simulink model "heat_transfer"  (R2021b)
settings: Solver=VariableStepAuto  StartTime=0.0  StopTime=10.0  RelTol=1e-3
libraries: fl_lib x21, nesl_utility x1
settings Model: Creator=310611102  LastModifiedBy=310611102

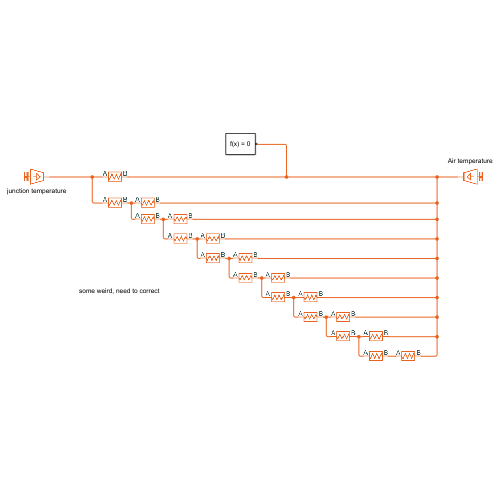
[thumbnail: Simulink's stored preview of the top-level diagram]
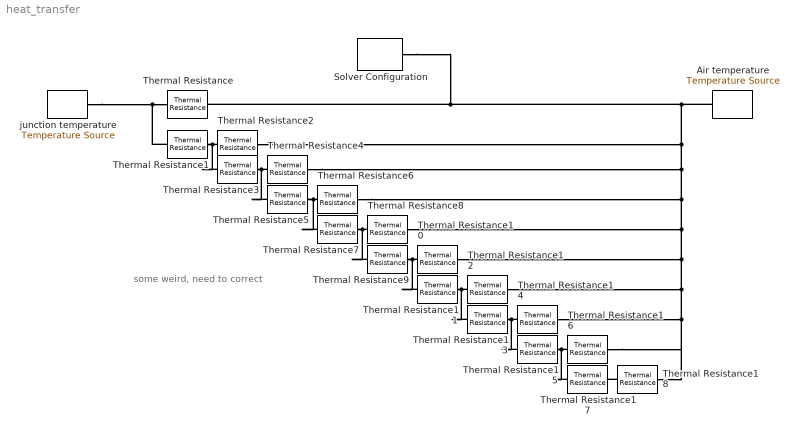
== system heat_transfer ==
  note: some weird, need to correct
  Air temperature : fl_lib/Thermal/Thermal Sources/Temperature Source  temperature=273.15+30 K
  Solver Configuration : nesl_utility/Solver Configuration  PhysicalDomain=network_engine_domain  SubClassName=solver  LeftPortType=input  RightPortType=generic  Tones=[]  Harmonics=[]  SimulateNoise=off  Profile=off  UseLocalSampling=off  EnableSwitchedLinearOptims=on  FrequencyDomain=off  UseCCode=off  RelTol=0.001  AbsTol=1e-06  MinStep=1e-09  ToWorkspace=off  RevertToSquareIcSolve=off  NumHomotopyIterations=100  PhasorMode=off  PhasorModeNumHarmonics=1  DoDC=off  ResidualTolerance=1e-09  UseLocalSolver=off  LocalSolverChoice=NE_BACKWARD_EULER_ADVANCER  LocalSolverSampleTime=0.001  DoFixedCost=off  MaxNonlinIter=3  MaxModeIter=2  ComputeImpulses=off  ImpulseIterations=2  LinearAlgebra=auto  EquationFormulation=NE_TIME_EF  DelaysMemoryBudget=1024  AutomaticFiltering=on  FilteringTimeConstant=0.001  PartitionStorageMethod=AS_NEEDED  PartitionMemoryBudget=1024  PartitionMethod=ROBUST
      settings: SourceProductBaseCode=PW,SS
  Thermal Resistance : fl_lib/Thermal/Thermal Elements/Thermal Resistance  resistance=Rchip_air K/W  T_specify=off  T_priority=None  T=0 K  T_nominal_specify=off  T_nominal_unit=K  T_nominal_value=1  Q_specify=off  Q_priority=None  Q=0 W  Q_nominal_specify=off  Q_nominal_unit=W  Q_nominal_value=1
      settings: SourceProductBaseCode=SS
  Thermal Resistance1 : fl_lib/Thermal/Thermal Elements/Thermal Resistance  resistance=Rchip_re1 K/W  T_specify=off  T_priority=None  T=0 K  T_nominal_specify=off  T_nominal_unit=K  T_nominal_value=1  Q_specify=off  Q_priority=None  Q=0 W  Q_nominal_specify=off  Q_nominal_unit=W  Q_nominal_value=1
      settings: SourceProductBaseCode=SS
  Thermal Resistance10 : fl_lib/Thermal/Thermal Elements/Thermal Resistance  resistance=Rfr45_air K/W  T_specify=off  T_priority=None  T=0 K  T_nominal_specify=off  T_nominal_unit=K  T_nominal_value=1  Q_specify=off  Q_priority=None  Q=0 W  Q_nominal_specify=off  Q_nominal_unit=W  Q_nominal_value=1
      settings: SourceProductBaseCode=SS
  Thermal Resistance11 : fl_lib/Thermal/Thermal Elements/Thermal Resistance  resistance=Rfr45_cop6 K/W  T_specify=off  T_priority=None  T=0 K  T_nominal_specify=off  T_nominal_unit=K  T_nominal_value=1  Q_specify=off  Q_priority=None  Q=0 W  Q_nominal_specify=off  Q_nominal_unit=W  Q_nominal_value=1
      settings: SourceProductBaseCode=SS
  Thermal Resistance12 : fl_lib/Thermal/Thermal Elements/Thermal Resistance  resistance=Rcop6_air K/W  T_specify=off  T_priority=None  T=0 K  T_nominal_specify=off  T_nominal_unit=K  T_nominal_value=1  Q_specify=off  Q_priority=None  Q=0 W  Q_nominal_specify=off  Q_nominal_unit=W  Q_nominal_value=1
      settings: SourceProductBaseCode=SS
  Thermal Resistance13 : fl_lib/Thermal/Thermal Elements/Thermal Resistance  resistance=Rcop6_fr47 K/W  T_specify=off  T_priority=None  T=0 K  T_nominal_specify=off  T_nominal_unit=K  T_nominal_value=1  Q_specify=off  Q_priority=None  Q=0 W  Q_nominal_specify=off  Q_nominal_unit=W  Q_nominal_value=1
      settings: SourceProductBaseCode=SS
  Thermal Resistance14 : fl_lib/Thermal/Thermal Elements/Thermal Resistance  resistance=Rfr47_air K/W  T_specify=off  T_priority=None  T=0 K  T_nominal_specify=off  T_nominal_unit=K  T_nominal_value=1  Q_specify=off  Q_priority=None  Q=0 W  Q_nominal_specify=off  Q_nominal_unit=W  Q_nominal_value=1
      settings: SourceProductBaseCode=SS
  Thermal Resistance15 : fl_lib/Thermal/Thermal Elements/Thermal Resistance  resistance=Rfr47_cop8 K/W  T_specify=off  T_priority=None  T=0 K  T_nominal_specify=off  T_nominal_unit=K  T_nominal_value=1  Q_specify=off  Q_priority=None  Q=0 W  Q_nominal_specify=off  Q_nominal_unit=W  Q_nominal_value=1
      settings: SourceProductBaseCode=SS
  Thermal Resistance16 : fl_lib/Thermal/Thermal Elements/Thermal Resistance  resistance=Rcop8_air K/W  T_specify=off  T_priority=None  T=0 K  T_nominal_specify=off  T_nominal_unit=K  T_nominal_value=1  Q_specify=off  Q_priority=None  Q=0 W  Q_nominal_specify=off  Q_nominal_unit=W  Q_nominal_value=1
      settings: SourceProductBaseCode=SS
  Thermal Resistance17 : fl_lib/Thermal/Thermal Elements/Thermal Resistance  resistance=Rcop8_re9 K/W  T_specify=off  T_priority=None  T=0 K  T_nominal_specify=off  T_nominal_unit=K  T_nominal_value=1  Q_specify=off  Q_priority=None  Q=0 W  Q_nominal_specify=off  Q_nominal_unit=W  Q_nominal_value=1
      settings: SourceProductBaseCode=SS
  Thermal Resistance18 : fl_lib/Thermal/Thermal Elements/Thermal Resistance  resistance=Rre9_air K/W  T_specify=off  T_priority=None  T=0 K  T_nominal_specify=off  T_nominal_unit=K  T_nominal_value=1  Q_specify=off  Q_priority=None  Q=0 W  Q_nominal_specify=off  Q_nominal_unit=W  Q_nominal_value=1
      settings: SourceProductBaseCode=SS
  Thermal Resistance2 : fl_lib/Thermal/Thermal Elements/Thermal Resistance  resistance=Rre1_air K/W  T_specify=off  T_priority=None  T=0 K  T_nominal_specify=off  T_nominal_unit=K  T_nominal_value=1  Q_specify=off  Q_priority=None  Q=0 W  Q_nominal_specify=off  Q_nominal_unit=W  Q_nominal_value=1
      settings: SourceProductBaseCode=SS
  Thermal Resistance3 : fl_lib/Thermal/Thermal Elements/Thermal Resistance  resistance=Rre1_cop2 K/W  T_specify=off  T_priority=None  T=0 K  T_nominal_specify=off  T_nominal_unit=K  T_nominal_value=1  Q_specify=off  Q_priority=None  Q=0 W  Q_nominal_specify=off  Q_nominal_unit=W  Q_nominal_value=1
      settings: SourceProductBaseCode=SS
  Thermal Resistance4 : fl_lib/Thermal/Thermal Elements/Thermal Resistance  resistance=Rcop2_air K/W  T_specify=off  T_priority=None  T=0 K  T_nominal_specify=off  T_nominal_unit=K  T_nominal_value=1  Q_specify=off  Q_priority=None  Q=0 W  Q_nominal_specify=off  Q_nominal_unit=W  Q_nominal_value=1
      settings: SourceProductBaseCode=SS
  Thermal Resistance5 : fl_lib/Thermal/Thermal Elements/Thermal Resistance  resistance=Rcop2_fr43 K/W  T_specify=off  T_priority=None  T=0 K  T_nominal_specify=off  T_nominal_unit=K  T_nominal_value=1  Q_specify=off  Q_priority=None  Q=0 W  Q_nominal_specify=off  Q_nominal_unit=W  Q_nominal_value=1
      settings: SourceProductBaseCode=SS
  Thermal Resistance6 : fl_lib/Thermal/Thermal Elements/Thermal Resistance  resistance=Rfr43_air K/W  T_specify=off  T_priority=None  T=0 K  T_nominal_specify=off  T_nominal_unit=K  T_nominal_value=1  Q_specify=off  Q_priority=None  Q=0 W  Q_nominal_specify=off  Q_nominal_unit=W  Q_nominal_value=1
      settings: SourceProductBaseCode=SS
  Thermal Resistance7 : fl_lib/Thermal/Thermal Elements/Thermal Resistance  resistance=Rfr43_cop4 K/W  T_specify=off  T_priority=None  T=0 K  T_nominal_specify=off  T_nominal_unit=K  T_nominal_value=1  Q_specify=off  Q_priority=None  Q=0 W  Q_nominal_specify=off  Q_nominal_unit=W  Q_nominal_value=1
      settings: SourceProductBaseCode=SS
  Thermal Resistance8 : fl_lib/Thermal/Thermal Elements/Thermal Resistance  resistance=Rcop4_air K/W  T_specify=off  T_priority=None  T=0 K  T_nominal_specify=off  T_nominal_unit=K  T_nominal_value=1  Q_specify=off  Q_priority=None  Q=0 W  Q_nominal_specify=off  Q_nominal_unit=W  Q_nominal_value=1
      settings: SourceProductBaseCode=SS
  Thermal Resistance9 : fl_lib/Thermal/Thermal Elements/Thermal Resistance  resistance=Rcop4_fr45 K/W  T_specify=off  T_priority=None  T=0 K  T_nominal_specify=off  T_nominal_unit=K  T_nominal_value=1  Q_specify=off  Q_priority=None  Q=0 W  Q_nominal_specify=off  Q_nominal_unit=W  Q_nominal_value=1
      settings: SourceProductBaseCode=SS
  junction temperature : fl_lib/Thermal/Thermal Sources/Temperature Source  temperature=273.15+100 K
  connections:
  Thermal Resistance2/LConn1 -- Thermal Resistance3/LConn1 -- Thermal Resistance1/RConn1
  Thermal Resistance1/LConn1 -- junction temperature/LConn1 -- Thermal Resistance/LConn1
  Air temperature/LConn1 -- Thermal Resistance2/RConn1 -- Thermal Resistance4/RConn1 -- Thermal Resistance6/RConn1 -- Thermal Resistance8/RConn1 -- Thermal Resistance10/RConn1 -- Thermal Resistance12/RConn1 -- Thermal Resistance14/RConn1 -- Thermal Resistance16/RConn1 -- Thermal Resistance18/RConn1 -- Solver Configuration/RConn1 -- Thermal Resistance/RConn1
  Thermal Resistance4/LConn1 -- Thermal Resistance5/LConn1 -- Thermal Resistance3/RConn1
  Thermal Resistance6/LConn1 -- Thermal Resistance7/LConn1 -- Thermal Resistance5/RConn1
  Thermal Resistance8/LConn1 -- Thermal Resistance9/LConn1 -- Thermal Resistance7/RConn1
  Thermal Resistance10/LConn1 -- Thermal Resistance11/LConn1 -- Thermal Resistance9/RConn1
  Thermal Resistance12/LConn1 -- Thermal Resistance13/LConn1 -- Thermal Resistance11/RConn1
  Thermal Resistance14/LConn1 -- Thermal Resistance15/LConn1 -- Thermal Resistance13/RConn1
  Thermal Resistance16/LConn1 -- Thermal Resistance17/LConn1 -- Thermal Resistance15/RConn1
  Thermal Resistance18/LConn1 -- Thermal Resistance17/RConn1
